simulink model "APContinuousSimulink"  (R2023b)
settings: Solver=VariableStepAuto  StartTime=0.0  StopTime=Tsim  RelTol=1e-3
values from neighbouring files (symbols this model uses):
  Aprime = T^(-1)*A*T    [APContinuous.m]
  Bprime = T^(-1)*B    [APContinuous.m]
  denp = [3 1]    [APContinuous.m]
  h = 6.5    [APContinuous.m]
  I = eye(size(A))    [APContinuous.m]
  K = 6*(-A)    [APContinuous.m]
  kr = (Cprime*((Bprime*K-Aprime)^(-1))*Bprime)^(-1)    [APContinuous.m]
  nump = [0 2]    [APContinuous.m]
  s = tf('s')    [APContinuous.m]
undefined symbols (not defined in the file or in its folder): A, B
libraries: cstblocks x16
settings Model: Creator=klysm  LastModifiedBy=klysm

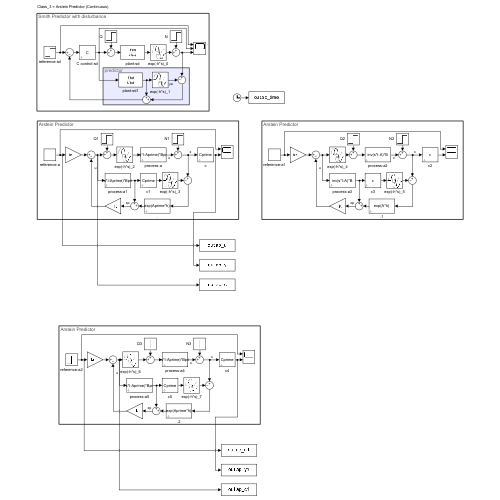
[thumbnail: Simulink's stored preview of the top-level diagram]
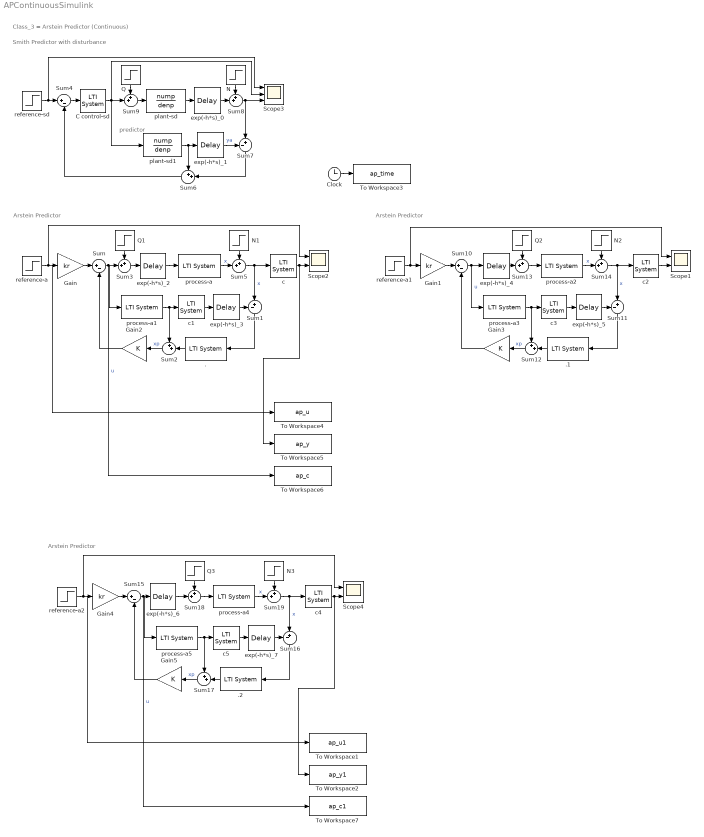
== system APContinuousSimulink ==
  note: Class_3 = Arstein Predictor (Continuous)
  note: Arstein Predictor
  note: Smith Predictor with disturbance
  note: predictor
  note: Arstein Predictor
  note: Arstein Predictor
  . : cstblocks/LTI System  sys=exp(Aprime*h)  IC=[]  PadeOrder=0
  .1 : cstblocks/LTI System  sys=exp(A*h)  IC=[]  PadeOrder=0
  .2 : cstblocks/LTI System  sys=exp(Aprime*h)  IC=[]  PadeOrder=0
  C control-sd : cstblocks/LTI System  sys=C  IC=[]  PadeOrder=0
  Clock : Clock
  Gain : Gain  Gain=kr
  Gain1 : Gain  Gain=kr
  Gain2 : Gain  Gain=K
  Gain3 : Gain  Gain=K
  Gain4 : Gain  Gain=kr
  Gain5 : Gain  Gain=K
  N : Step  Time=20  After=0.2  SampleTime=0
  N1 : Step  Time=0  After=0  SampleTime=0
  N2 : Step  Time=20  After=0.2  SampleTime=0
  N3 : Step  Time=20  After=0.2  SampleTime=0
  Q : Step  Time=10  After=0.2  SampleTime=0
  Q1 : Step  Time=0  After=0  SampleTime=0
  Q2 : Step  Time=10  After=0.2  SampleTime=0
  Q3 : Step  Time=10  After=0.2  SampleTime=0
  Scope1 : Scope  NumInputPorts=2
  Scope2 : Scope  NumInputPorts=2
  Scope3 : Scope  NumInputPorts=3
  Scope4 : Scope  NumInputPorts=2
  Sum{,4,10,15} (4 alike) : Sum  Inputs=|+-
  Sum{1,7,11,16} (4 alike) : Sum  Inputs=-+|
  Sum{2..3,5..6,8..9,12..14,17..19} (12 alike) : Sum  Inputs=++|
  To Workspace1 : ToWorkspace  VariableName=ap_u1  SampleTime=-1
  To Workspace2 : ToWorkspace  VariableName=ap_y1  SampleTime=-1
  To Workspace3 : ToWorkspace  VariableName=ap_time  SampleTime=-1
  To Workspace4 : ToWorkspace  VariableName=ap_u  SampleTime=-1
  To Workspace5 : ToWorkspace  VariableName=ap_y  SampleTime=-1
  To Workspace6 : ToWorkspace  VariableName=ap_c  SampleTime=-1
  To Workspace7 : ToWorkspace  VariableName=ap_c1  SampleTime=-1
  c{,1,4..5} (4 alike) : cstblocks/LTI System  sys=Cprime  IC=[]  PadeOrder=0
  c2 : cstblocks/LTI System  sys=c  IC=[]  PadeOrder=0
  c3 : cstblocks/LTI System  sys=c  IC=[]  PadeOrder=0
  exp(-h*s)_{0..7} (8 alike) : TransportDelay  DelayTime=h
  plant-sd : TransferFcn  Numerator=nump  Denominator=denp
  plant-sd1 : TransferFcn  Numerator=nump  Denominator=denp
  process-a{,1,4..5} (4 alike) : cstblocks/LTI System  sys=inv(s*I-Aprime)*Bprime  IC=[]  PadeOrder=0
  process-a2 : cstblocks/LTI System  sys=inv(s*I-A)*B  IC=[]  PadeOrder=0
  process-a3 : cstblocks/LTI System  sys=inv(s*I-A)*B  IC=[]  PadeOrder=0
  reference-a : Step  Time=0  SampleTime=0
  reference-a1 : Step  Time=0  SampleTime=0
  reference-a2 : Step  Time=0  SampleTime=0
  reference-sd : Step  Time=0  SampleTime=0
  wires:
  Gain/1 -> Sum/1
  reference-a/1 -> To Workspace4/1, Scope2/1, Gain/1
  Sum/1 -> Sum3/2, process-a1/1, To Workspace6/1  "u"
  process-a1/1 -> c1/1, Sum2/1
  Sum5/1 -> c/1, Sum1/2  "x"
  exp(-h*s)_3/1 -> Sum1/1
  ./1 -> Sum2/2
  Sum1/1 -> ./1
  Sum2/1 -> Gain2/1  "xp"
  Gain2/1 -> Sum/2
  c/1 -> To Workspace5/1, Scope2/2
  c1/1 -> exp(-h*s)_3/1
  process-a/1 -> Sum5/2  "x"
  N1/1 -> Sum5/1
  Q/1 -> Sum9/1
  Sum8/1 -> Scope3/3, Sum7/2
  Sum9/1 -> plant-sd/1
  plant-sd1/1 -> Sum6/1, exp(-h*s)_1/1
  Sum6/1 -> Sum4/2
  Sum7/1 -> Sum6/2
  exp(-h*s)_0/1 -> Sum8/2
  exp(-h*s)_1/1 -> Sum7/1  "ya"
  reference-sd/1 -> Scope3/1, Sum4/1
  C control-sd/1 -> Sum9/2, Scope3/2, plant-sd1/1
  plant-sd/1 -> exp(-h*s)_0/1
  N/1 -> Sum8/1
  Sum4/1 -> C control-sd/1
  exp(-h*s)_2/1 -> process-a/1
  Sum3/1 -> exp(-h*s)_2/1
  Q1/1 -> Sum3/1
  Gain1/1 -> Sum10/1
  c3/1 -> exp(-h*s)_5/1
  exp(-h*s)_4/1 -> Sum13/2
  process-a2/1 -> Sum14/2  "x"
  N2/1 -> Sum14/1
  .1/1 -> Sum12/2
  reference-a1/1 -> Scope1/1, Gain1/1
  Gain3/1 -> Sum10/2
  exp(-h*s)_5/1 -> Sum11/1
  Sum14/1 -> c2/1, Sum11/2  "x"
  Sum10/1 -> exp(-h*s)_4/1, process-a3/1  "u"
  Sum11/1 -> .1/1
  process-a3/1 -> c3/1, Sum12/1
  c2/1 -> Scope1/2
  Sum12/1 -> Gain3/1  "xp"
  Sum13/1 -> process-a2/1
  Q2/1 -> Sum13/1
  Clock/1 -> To Workspace3/1
  .2/1 -> Sum17/2
  Sum19/1 -> c4/1, Sum16/2  "x"
  c5/1 -> exp(-h*s)_7/1
  Q3/1 -> Sum18/1
  Sum18/1 -> process-a4/1
  N3/1 -> Sum19/1
  Sum17/1 -> Gain5/1  "xp"
  c4/1 -> To Workspace2/1, Scope4/2
  Sum16/1 -> .2/1
  process-a4/1 -> Sum19/2  "x"
  Sum15/1 -> process-a5/1, exp(-h*s)_6/1, To Workspace7/1  "u"
  Gain5/1 -> Sum15/2
  reference-a2/1 -> To Workspace1/1, Scope4/1, Gain4/1
  process-a5/1 -> c5/1, Sum17/1
  exp(-h*s)_7/1 -> Sum16/1
  Gain4/1 -> Sum15/1
  exp(-h*s)_6/1 -> Sum18/2
